simulink model "Topo_5Gsimulink_handover"  (R2022a)
settings: Solver=VariableStepAuto  StartTime=0.0  StopTime=10.0  RelTol=1e-3
settings Model: Creator=ASUS  LastModifiedBy=ASUS
settings DataIOCC: SaveFormat=Array  ReturnWorkspaceOutputs=off  LoggingToFile=on

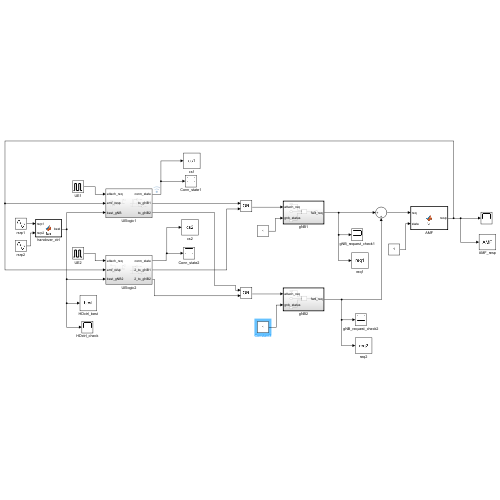
[thumbnail: Simulink's stored preview of the top-level diagram]
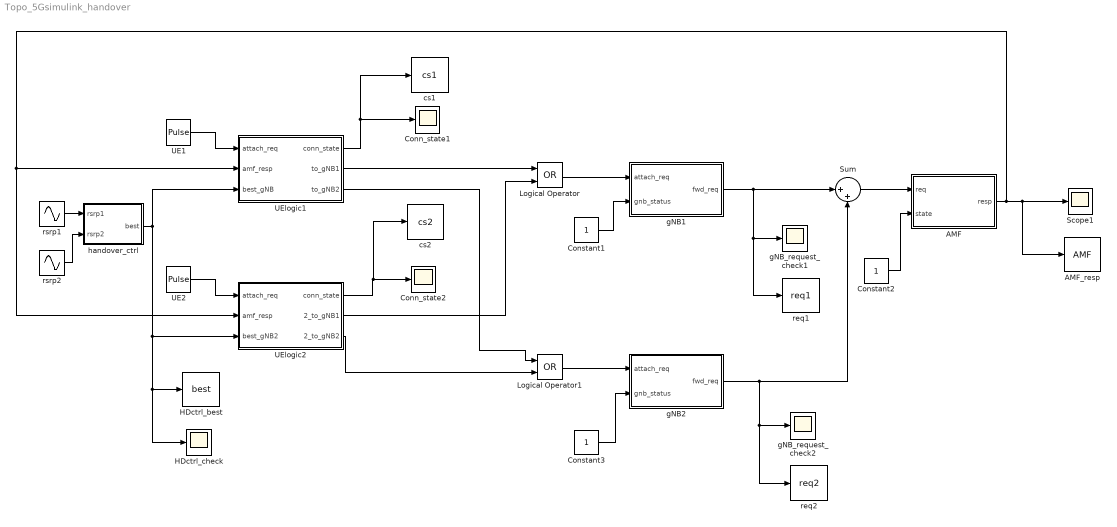
== system Topo_5Gsimulink_handover ==
  AMF : MATLAB Function  TreatAsAtomicUnit=on
  AMF_resp : ToWorkspace  VariableName=AMF  SaveFormat=Structure With Time  SampleTime=-1
      settings: Save2DSignal=2-D array (concatenate along first dimension)
  Conn_state1 : Scope
  Conn_state2 : Scope
  Constant1 : Constant
  Constant2 : Constant
  Constant3 : Constant
  HDctrl_best : ToWorkspace  VariableName=best  SaveFormat=Structure With Time  SampleTime=-1
      settings: Save2DSignal=2-D array (concatenate along first dimension)
  HDctrl_check : Scope
  Logical Operator : Logic  Operator=OR  AllPortsSameDT=off  OutDataTypeStr=boolean
  Logical Operator1 : Logic  Operator=OR  AllPortsSameDT=off  OutDataTypeStr=boolean
  Scope1 : Scope
  Sum : Sum  Inputs=|++
  UE1 : DiscretePulseGenerator  PulseType=Time based  PulseWidth=50
  UE2 : DiscretePulseGenerator  PulseType=Time based  PulseWidth=50
  UElogic1 : Subsystem
  UElogic2 : Subsystem
  cs1 : ToWorkspace  VariableName=cs1  SaveFormat=Structure With Time  SampleTime=-1
      settings: Save2DSignal=2-D array (concatenate along first dimension)
  cs2 : ToWorkspace  VariableName=cs2  SaveFormat=Structure With Time  SampleTime=-1
      settings: Save2DSignal=2-D array (concatenate along first dimension)
  gNB1 : Subsystem  TreatAsAtomicUnit=on
  gNB2 : Subsystem  TreatAsAtomicUnit=on
  gNB_request_check1 : Scope
  gNB_request_check2 : Scope
  handover_ctrl : MATLAB Function  TreatAsAtomicUnit=on
  req1 : ToWorkspace  VariableName=req1  SaveFormat=Structure With Time  SampleTime=-1
      settings: Save2DSignal=2-D array (concatenate along first dimension)
  req2 : ToWorkspace  VariableName=req2  SaveFormat=Structure With Time  SampleTime=-1
      settings: Save2DSignal=2-D array (concatenate along first dimension)
  rsrp1 : Sin  Amplitude=30  Bias=60  Frequency=0.628  SampleTime=0
  rsrp2 : Sin  Amplitude=30  Bias=60  Frequency=0.628  Phase=3.1416  SampleTime=0
  wires:
  Constant1/1 -> gNB1/2(gnb_status)
  UElogic1/1(conn_state) -> cs1/1, Conn_state1/1
  Constant2/1 -> AMF/2(state)
  gNB1/1(" fwd_req") -> Sum/1, req1/1, gNB_request_check1/1
  UE2/1 -> UElogic2/1(attach_req)
  Constant3/1 -> gNB2/2(gnb_status)
  Sum/1 -> AMF/1(req)
  gNB2/1(" fwd_req") -> Sum/2, gNB_request_check2/1, req2/1
  UE1/1 -> UElogic1/1(attach_req)
  AMF/1(resp) -> UElogic2/2(amf_resp), UElogic1/2(amf_resp), AMF_resp/1, Scope1/1
  UElogic2/1(conn_state) -> cs2/1, Conn_state2/1
  rsrp1/1 -> handover_ctrl/1(rsrp1)
  rsrp2/1 -> handover_ctrl/2(rsrp2)
  handover_ctrl/1(best) -> UElogic2/3(best_gNB2), HDctrl_check/1, HDctrl_best/1, UElogic1/3(best_gNB)
  Logical Operator/1 -> gNB1/1(attach_req)
  UElogic1/2(to_gNB1) -> Logical Operator/1
  UElogic2/2(2_to_gNB1) -> Logical Operator/2
  Logical Operator1/1 -> gNB2/1(attach_req)
  UElogic2/3(2_to_gNB2) -> Logical Operator1/2
  UElogic1/3(to_gNB2) -> Logical Operator1/1

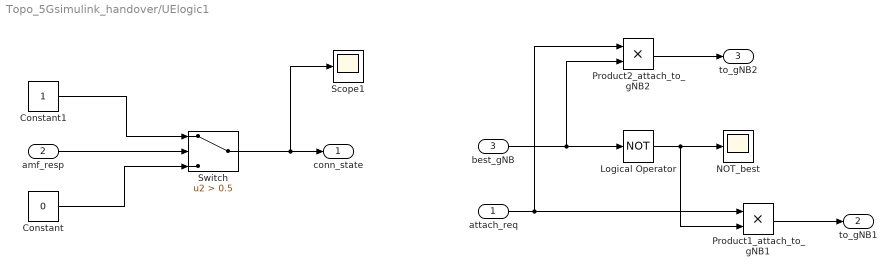
== system Topo_5Gsimulink_handover/UElogic1 ==
  attach_req : Inport
  amf_resp : Inport  Port=2
  best_gNB : Inport  Port=3
  Constant : Constant  Value=0
  Constant1 : Constant
  Logical Operator : Logic  Operator=NOT  AllPortsSameDT=off  OutDataTypeStr=boolean
  NOT_best : Scope
  Product1_attach_to_gNB1 : Product
  Product2_attach_to_gNB2 : Product
  Scope1 : Scope
  Switch : Switch  Criteria=u2 > Threshold  Threshold=0.5  SaturateOnIntegerOverflow=off  InputSameDT=off
  conn_state : Outport
  to_gNB1 : Outport  Port=2
  to_gNB2 : Outport  Port=3
  wires:
  Constant/1 -> Switch/3
  Switch/1 -> Scope1/1, conn_state/1
  amf_resp/1 -> Switch/2
  Constant1/1 -> Switch/1
  best_gNB/1 -> Product2_attach_to_gNB2/2, Logical Operator/1
  Logical Operator/1 -> NOT_best/1, Product1_attach_to_gNB1/2
  attach_req/1 -> Product2_attach_to_gNB2/1, Product1_attach_to_gNB1/1
  Product2_attach_to_gNB2/1 -> to_gNB2/1
  Product1_attach_to_gNB1/1 -> to_gNB1/1

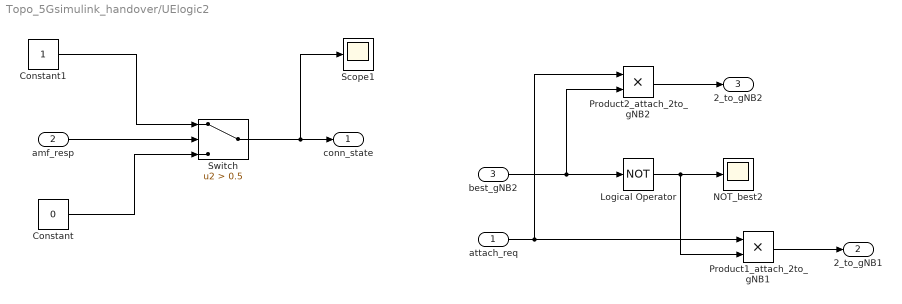
== system Topo_5Gsimulink_handover/UElogic2 ==
  attach_req : Inport
  amf_resp : Inport  Port=2
  best_gNB2 : Inport  Port=3
  Constant : Constant  Value=0
  Constant1 : Constant
  Logical Operator : Logic  Operator=NOT  AllPortsSameDT=off  OutDataTypeStr=boolean
  NOT_best2 : Scope
  Product1_attach_2to_gNB1 : Product
  Product2_attach_2to_gNB2 : Product
  Scope1 : Scope
  Switch : Switch  Criteria=u2 > Threshold  Threshold=0.5  SaturateOnIntegerOverflow=off  InputSameDT=off
  conn_state : Outport
  2_to_gNB1 : Outport  Port=2
  2_to_gNB2 : Outport  Port=3
  wires:
  Constant/1 -> Switch/3
  Switch/1 -> Scope1/1, conn_state/1
  amf_resp/1 -> Switch/2
  Constant1/1 -> Switch/1
  best_gNB2/1 -> Product2_attach_2to_gNB2/2, Logical Operator/1
  Logical Operator/1 -> NOT_best2/1, Product1_attach_2to_gNB1/2
  Product2_attach_2to_gNB2/1 -> 2_to_gNB2/1
  attach_req/1 -> Product2_attach_2to_gNB2/1, Product1_attach_2to_gNB1/1
  Product1_attach_2to_gNB1/1 -> 2_to_gNB1/1

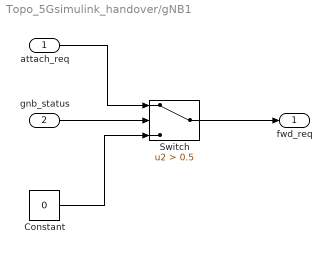
== system Topo_5Gsimulink_handover/gNB1 ==
  attach_req : Inport
  gnb_status : Inport  Port=2
  Constant : Constant  Value=0
  Switch : Switch  Criteria=u2 > Threshold  Threshold=0.5  SaturateOnIntegerOverflow=off  InputSameDT=off
  " fwd_req" : Outport
  wires:
  attach_req/1 -> Switch/1
  gnb_status/1 -> Switch/2
  Constant/1 -> Switch/3
  Switch/1 -> " fwd_req"/1

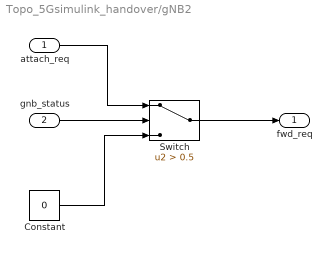
== system Topo_5Gsimulink_handover/gNB2 ==
  attach_req : Inport
  gnb_status : Inport  Port=2
  Constant : Constant  Value=0
  Switch : Switch  Criteria=u2 > Threshold  Threshold=0.5  SaturateOnIntegerOverflow=off  InputSameDT=off
  " fwd_req" : Outport
  wires:
  attach_req/1 -> Switch/1
  gnb_status/1 -> Switch/2
  Constant/1 -> Switch/3
  Switch/1 -> " fwd_req"/1

== matlab function Topo_5Gsimulink_handover/handover_ctrl ==
  data: rsrp1 input; best output; rsrp2 input
function best = fcn(rsrp1, rsrp2)
% best = 0 → 选 gNB1
% best = 1 → 选 gNB2
delta = 3;                % 切换阈值 3 dB
if rsrp2 - rsrp1 > delta
    best = 1;
else
    best = 0;
end

== matlab function Topo_5Gsimulink_handover/AMF ==
  data: req input; resp output; state input
function resp = fcn(req, state)
%#codegen
% req   : 1 表示 UE attach 请求已到 gNB
% state : 0=reject, 1=accept, 2=fallback
% resp  : 0=失败, 1=成功, 2=应急

% 没有请求时，直接输出 0
if req == 0
    resp = 0;
    return;
end

switch state
    case 1      % 接受
        resp = 1;
    case 2      % 应急 / fallback
        resp = 2;
    otherwise   % 拒绝
        resp = 0;
end
